simulink subsystem "AngularRateTransform"  (R2022a)
settings: Solver=VariableStepAuto  StartTime=0.0  StopTime=10.0  RelTol=1e-3
settings Model: Creator=charl  LastModifiedBy=charl

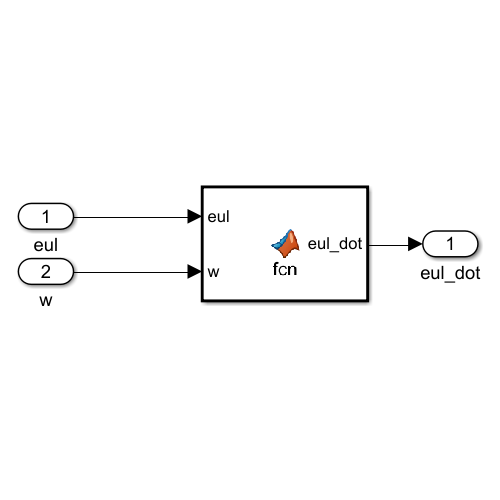
[thumbnail: Simulink's stored preview of the top-level diagram]
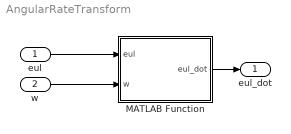
== system AngularRateTransform ==
  eul : Inport
  w : Inport  Port=2
  MATLAB Function : MATLAB Function  TreatAsAtomicUnit=on
  eul_dot : Outport
  wires:
  MATLAB Function/1(eul_dot) -> eul_dot/1
  w/1 -> MATLAB Function/2(w)
  eul/1 -> MATLAB Function/1(eul)

== matlab function AngularRateTransform/MATLAB Function ==
  data: eul input; eul_dot output; w input
function eul_dot = fcn(eul, w)

eul_dot = omega2euler(eul, w);
